simulink library "sm_forklift_lib"  (R2026a)
settings: Solver=VariableStepAuto
undefined symbols (not defined in the file): ForkliftParams, X, Y, Z
libraries: sm_lib x3, $bdroot x2, fl_lib x1, nesl_utility x1
Description:
  | Copyright 2025-2026 The MathWorks, Inc.
settings Model: Creator=smiller  LastModifiedBy=smiller

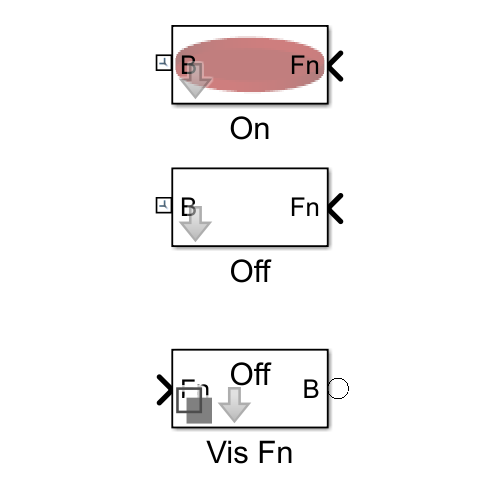
[thumbnail: Simulink's stored preview of the top-level diagram]
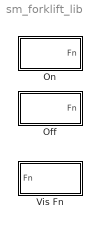
== system sm_forklift_lib ==
  Off : Subsystem  mask{vis_max_rad=0.5, vis_min_rad=1e-3, tFilt=0.01, NtoRad=0.5, vis_offset=ForkliftParams.groundContact.rearTireRad-0.02}
      mask prompts: vis_max_rad "Max Radius (m)"; vis_min_rad "Min Radius (m)"; tFilt "Filter constant (sec)"; NtoRad "Force to Radius gain (m/N)"; vis_offset "Vis Offset from Axle (m)"
      settings: PortSchema="{\"entries\":[{\"content\":{\"sides\":[{\"content\":{\"connectorIds\":[\"LConn1\"]},\"type\":\"ConnectorPlacement.EquallySpacedRectSide\",\"uuid\":\"e24539ec-9354-402f-b547-7a2c9229cda4\"},{\"content\":{\"connectorIds\":[\"In1\"],\"side\":\"RIGHT\"},\"type\":\"ConnectorPlacement.EquallySpacedRectSide\",\"uuid\":\"5a444927-40bb-43e7-bc77-0c66791634d2\"},{\"content\":{\"side\":\"TOP\"},\"type\":\"ConnectorPlacement.EquallySpacedRectSide\",\"uuid\":\"8ef1afb6-2e0f-4bae-985a-572cd4673b5a\"}]},\"type\":\"ConnectorPlacement.EquallySpacedConnector\",\"uuid\":\"b1ef4159-b9a3-4446-870d-8bfbaec2bcb1\"}],\"packageUris\":[\"http://schema.mathworks.com/mf0/Connector/R2020b\"],\"version\":\"1.0\"}"
  On : Subsystem  mask{vis_max_rad=0.5, vis_min_rad=1e-3, tFilt=0.01, NtoRad=0.5, vis_offset=ForkliftParams.groundContact.rearTireRad-0.02}
      mask prompts: vis_max_rad "Max Radius (m)"; vis_min_rad "Min Radius (m)"; tFilt "Filter constant (sec)"; NtoRad "Force to Radius gain (m/N)"; vis_offset "Vis Offset from Axle (m)"
      settings: PortSchema="{\"entries\":[{\"content\":{\"sides\":[{\"content\":{\"connectorIds\":[\"LConn1\"]},\"type\":\"ConnectorPlacement.EquallySpacedRectSide\",\"uuid\":\"e24539ec-9354-402f-b547-7a2c9229cda4\"},{\"content\":{\"connectorIds\":[\"In1\"],\"side\":\"RIGHT\"},\"type\":\"ConnectorPlacement.EquallySpacedRectSide\",\"uuid\":\"5a444927-40bb-43e7-bc77-0c66791634d2\"},{\"content\":{\"side\":\"TOP\"},\"type\":\"ConnectorPlacement.EquallySpacedRectSide\",\"uuid\":\"8ef1afb6-2e0f-4bae-985a-572cd4673b5a\"}]},\"type\":\"ConnectorPlacement.EquallySpacedConnector\",\"uuid\":\"b1ef4159-b9a3-4446-870d-8bfbaec2bcb1\"}],\"packageUris\":[\"http://schema.mathworks.com/mf0/Connector/R2020b\"],\"version\":\"1.0\"}"
      mask Display: image('sm_forklift_vis_normalForce_image.png')
  Vis Fn : Subsystem  Variant=on  VariantControlMode=label  VariantControl=Vis Fn R  LabelModeActiveChoice=Off  mask{popup_fnVis_onOff=Off, vis_offset=(ForkliftParams.groundContact.frontTireRad-0.02)}
      mask prompts: popup_fnVis_onOff "Normal Force Visualization"; vis_offset "Visualization Vertical Offset (m)"
      mask init:
      | bh = gcb;
      | set_param(bh,'LabelModeActiveChoice',get_param(bh,'popup_fnVis_OnOff'));
      settings: PortSchema="{\"entries\":[{\"content\":{\"sides\":[{\"content\":{\"connectorIds\":[\"LConn1\"]},\"type\":\"ConnectorPlacement.EquallySpacedRectSide\",\"uuid\":\"e24539ec-9354-402f-b547-7a2c9229cda4\"},{\"content\":{\"connectorIds\":[\"In1\"],\"side\":\"RIGHT\"},\"type\":\"ConnectorPlacement.EquallySpacedRectSide\",\"uuid\":\"5a444927-40bb-43e7-bc77-0c66791634d2\"},{\"content\":{\"side\":\"TOP\"},\"type\":\"ConnectorPlacement.EquallySpacedRectSide\",\"uuid\":\"8ef1afb6-2e0f-4bae-985a-572cd4673b5a\"}]},\"type\":\"ConnectorPlacement.EquallySpacedConnector\",\"uuid\":\"b1ef4159-b9a3-4446-870d-8bfbaec2bcb1\"}],\"packageUris\":[\"http://schema.mathworks.com/mf0/Connector/R2020b\"],\"version\":\"1.0\"}"
      mask TypeOptions popup_fnVis_onOff: On | Off

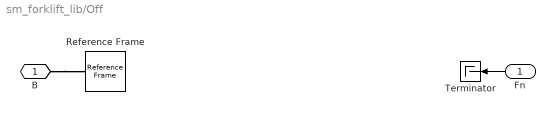
== system sm_forklift_lib/Off ==
  Fn : Inport
  Reference Frame : sm_lib/Frames and Transforms/Reference Frame
  Terminator : Terminator
  B : PMIOPort  Side=Left
  wires:
  Fn/1 -> Terminator/1
  connections:
  B/RConn1 -- Reference Frame/RConn1

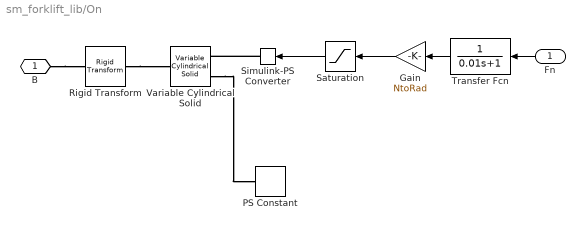
== system sm_forklift_lib/On ==
  Fn : Inport
  Gain : Gain  Gain=NtoRad
  PS Constant : fl_lib/Physical Signals/Sources/PS Constant  constant=0.01 kg
  Rigid Transform : sm_lib/Frames and Transforms/Rigid Transform  RotationMethod=StandardAxis  FollAlignAxisA=+X  BaseAlignAxisA=+Y  FollAlignAxisB=+Y  BaseAlignAxisB=+Z  RotationStandardAxis=+Y  RotationAngle=90  RotationAngleUnits=deg  RotationArbitraryAxis=[0 0 1]  RotationSequenceAxes=FollowerAxes  RotationSequence=XYX  RotationSequenceAngles=[0 0 0]  RotationSequenceAnglesUnits=deg  RotationMatrix=[1 0 0;0 1 0;0 0 1]  Quaternion=[1 0 0 0]  TranslationMethod=StandardAxis  TranslationCartesianOffset=[0 0 0]  TranslationCartesianOffsetUnits=m  TranslationStandardAxis=-X  TranslationStandardOffset=vis_offset  TranslationStandardOffsetUnits=m  TranslationROffset=0  TranslationROffsetUnits=m  TranslationThetaOffset=0  TranslationThetaOffsetUnits=deg  TranslationZOffset=0  TranslationZOffsetUnits=m
  Saturation : Saturate  UpperLimit=vis_max_rad  LowerLimit=vis_min_rad  ZeroCross=off  OutMin=1e-3  OutMax=1
  Simulink-PS Converter : nesl_utility/Simulink-PS Converter  PhysicalDomain=network_engine_domain  SubClassName=ps_input  LeftPortType=input  RightPortType=output  PseudoPeriodic=off  Frequencies=[]  NoiseDistribution=none  NoiseParameters=[]  Unit=m  AffineConversion=off  FilteringAndDerivatives=provide  SimscapeFilterOrder=1  InputFilterTimeConstant=0.001  UdotUserProvided=0
  Transfer Fcn : TransferFcn  Denominator=[0.01 1]
  Variable Cylindrical Solid : sm_lib/Body Elements/Variable Mass/Variable Cylindrical Solid  ComputedVariable=Density  RadiusType=ProvidedByInput  Radius=1  RadiusUnits=m  LengthType=Constant  Length=0.02  LengthUnits=m  DensityType=Constant  Density=1000  DensityUnits=kg/m^3  MassType=ProvidedByInput  Mass=1  MassUnits=kg  SenseRadius=off  SenseLength=off  SenseDensity=off  SenseMass=off  SenseCenterOfMass=off  SenseInertiaMatrix=off  GraphicType=FromGeometry  MarkerShape=Sphere  MarkerSize=10  GraphicVisPropType=SimpleVisualProperties  GraphicDiffuseColor=[1 0 0]  GraphicOpacity=0.3  GraphicSpecularColor=[0.5 0.5 0.5 1.0]  GraphicAmbientColor=[0.15 0.15 0.15 1.0]  GraphicEmissiveColor=[0.0 0.0 0.0 1.0]  GraphicShininess=75
  B : PMIOPort  Side=Left
  wires:
  Fn/1 -> Transfer Fcn/1
  Transfer Fcn/1 -> Gain/1
  Saturation/1 -> Simulink-PS Converter/1
  Gain/1 -> Saturation/1
  connections:
  Rigid Transform/RConn1 -- Variable Cylindrical Solid/RConn1
  B/RConn1 -- Rigid Transform/LConn1
  Variable Cylindrical Solid/LConn2 -- PS Constant/RConn1
  Simulink-PS Converter/RConn1 -- Variable Cylindrical Solid/LConn1

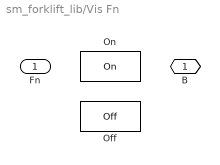
== system sm_forklift_lib/Vis Fn ==
  Fn : Inport
  Off : $bdroot/Off  VariantControl=Off  vis_max_rad=0.5  vis_min_rad=1e-3  tFilt=0.01  NtoRad=0.5  vis_offset=ForkliftParams.groundContact.rearTireRad-0.02
  On : $bdroot/On  VariantControl=On  vis_max_rad=0.5  vis_min_rad=1e-3  tFilt=0.01  NtoRad=ForkliftParams.FnVis.FtoRGain  vis_offset=vis_offset
  B : PMIOPort  Side=Left
